simulink model "SS_1029"  (R2014a)
settings: Solver=FixedStepDiscrete  StartTime=0.0  StopTime=5  FixedStep=0.0005  RelTol=1e-3
values from neighbouring files (symbols this model uses):
  APS_High_null = ecucoder_cal(APS_High_null)    [SS.m]
  APS_High_x = ecucoder_cal(APS_High_x)    [SS.m]
  APS_High_y = ecucoder_cal(APS_High_y)    [SS.m]
  APS_Low_null = ecucoder_cal(APS_Low_null)    [SS.m]
  APS_low_x = ecucoder_cal(APS_low_x)    [SS.m]
  APS_low_y = ecucoder_cal(APS_low_y)    [SS.m]
  BrakeSignal_cal = ecucoder_cal(BrakeSignal_cal)    [SS.m]
  CustomReduceFactor_cal = ecucoder_cal(CustomReduceFactor_cal)    [SS.m]
  Differential_cal = ecucoder_cal(Differential_cal)    [SS.m]
  LowSOCWarning_cal = ecucoder_cal(LowSOCWarning_cal)    [SS.m]
  MotorTemperatureHigh_cal = ecucoder_cal(MotorTemperatureHigh_cal)    [SS.m]
  MotorTemperatureLow_cal = ecucoder_cal(MotorTemperatureLow_cal)    [SS.m]
  OilPressure_x = ecucoder_cal(OilPressure_x)    [SS.m]
  OilPressure_y = ecucoder_cal(OilPressure_y)    [SS.m]
  PowerBias_cal = ecucoder_cal(PowerBias_cal)    [SS.m]
  SpeedLimitFactor_x = ecucoder_cal(SpeedLimitFactor_x)    [SS.m]
  SpeedLimitFactor_y = ecucoder_cal(SpeedLimitFactor_y)    [SS.m]
  TorqueLimitNegativ_cal = ecucoder_cal(TorqueLimitNegativ_cal)    [SS.m]
  TorqueLimitPositiv_cal = ecucoder_cal(TorqueLimitPositiv_cal)    [SS.m]
libraries: simulink x101, ec55xxlib x31
(part 1 of 3)
settings Model: Creator=BIT-Battery Group  LastModifiedBy=Administrator
settings OptimizationCC: InlineParams=on  InlineInvariantSignals=on  RollThreshold=9  StateBitsets=on  DataBitsets=on  UseTempVars=on  ZeroExternalMemoryAtStartup=off  ZeroInternalMemoryAtStartup=off  EfficientFloat2IntCast=on  OptimizeModelRefInitCode=on  LifeSpan=Inf
settings DebuggingCC: ConsistencyChecking=warning  MaxConsecutiveZCsMsg=warning  InheritedTsInSrcMsg=none  ModelReferenceExtraNoncontSigs=warning  SimStateOlderReleaseMsg=warning
settings HardwareCC: ProdLargestAtomicInteger=Long  ProdLargestAtomicFloat=Double  ProdIntDivRoundTo=Zero  ProdEndianess=BigEndian  ProdHWDeviceType=Freescale MPC5500
settings RTWCC: SystemTargetFile=ec55xx.tlc  MakeCommand=make_rtw optimized_fixed_point=1  GenerateMakefile=off  TemplateMakefile=ec55xx_lcc.tmf  PostCodeGenCommand=ec55xx_pst_s2(buildInfo)  Description=Target for EC55XX  GenerateReport=on  ProcessScript=ec55xx_make_rtw_hook  IncludeHyperlinkInReport=on  LaunchReport=on
settings CodeAppCC: IgnoreCustomStorageClasses=off
settings STFCustomTargetCC: ModelReferenceCompliant=off  ConcurrentExecutionCompliant=off  IncludeMdlTerminateFcn=off  GeneratePreprocessorConditionals=Use local settings  CombineOutputUpdateFcns=on  SuppressErrorStatus=on  ERTCustomFileBanners=on  SupportContinuousTime=off  SupportNonInlinedSFcns=off  MATLABClassNameForMDSCustomization=Simulink.SoftwareTarget.ERTCustomization  GRTInterface=off  SystemTargetFile=ec55xx.tlc
settings ERTTargetCC: GenerateSampleERTMain=off  ModelReferenceCompliant=off  IncludeMdlTerminateFcn=off  SuppressErrorStatus=on  GenerateASAP2=on  ERTSrcFileBannerTemplate=ec55xx_code_template.cgt  ERTHdrFileBannerTemplate=ec55xx_code_template.cgt  ERTDataSrcFileTemplate=ec55xx_code_template.cgt  ERTDataHdrFileTemplate=ec55xx_code_template.cgt  ERTCustomFileTemplate=ec55xx_file_process.tlc

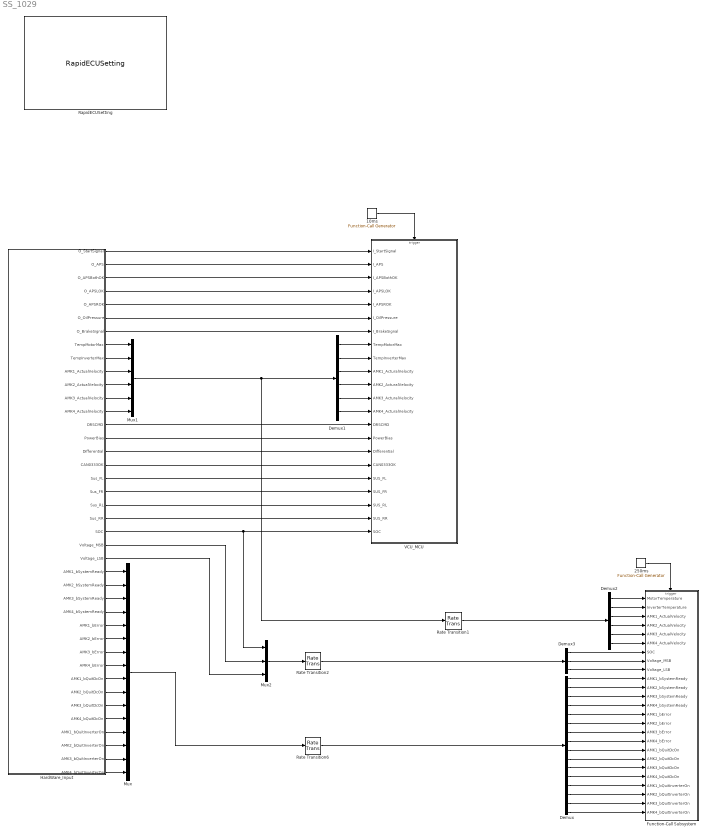
== system SS_1029 ==
  10ms : simulink/Ports & Subsystems/Function-Call Generator  sample_time=0.01  numberOfIterations=1
  250ms : simulink/Ports & Subsystems/Function-Call Generator  sample_time=0.25  numberOfIterations=1
  Demux : Demux  Outputs=16
  Demux1 : Demux  Outputs=6
  Demux2 : Demux  Outputs=6
  Demux3 : Demux  Outputs=3
  Function-Call Subsystem : Subsystem  TreatAsAtomicUnit=on
  HardWare_Input : Subsystem  TreatAsAtomicUnit=on
  Mux : Mux  Inputs=16
  Mux1 : Mux  Inputs=6
  Mux2 : Mux  Inputs=3
  RapidECUSetting : ec55xxlib/RapidECU_U2/RapidECUSetting
  Rate Transition1 : RateTransition  OutPortSampleTime=0.25
  Rate Transition2 : RateTransition  OutPortSampleTime=0.25
  Rate Transition6 : RateTransition  OutPortSampleTime=0.25
  VCU_MCU : Subsystem  TreatAsAtomicUnit=on
  wires:
  HardWare_Input/1(O_StartSignal) -> VCU_MCU/1(I_StartSignal)
  HardWare_Input/5(O_APSROK) -> VCU_MCU/5(I_APSROK)
  HardWare_Input/6(O_OilPressure) -> VCU_MCU/6(I_OilPressure)
  HardWare_Input/4(O_APSLOK) -> VCU_MCU/4(I_APSLOK)
  HardWare_Input/3(O_APSBothOK) -> VCU_MCU/3(I_APSBothOK)
  HardWare_Input/2(O_APS) -> VCU_MCU/2(I_APS)
  10ms/1 -> VCU_MCU/Trigger
  HardWare_Input/7(O_BrakeSignal) -> VCU_MCU/7(I_BrakeSignal)
  250ms/1 -> Function-Call Subsystem/Trigger
  HardWare_Input/22(SOC) -> Mux2/1, VCU_MCU/22(SOC)
  HardWare_Input/14(DRSCMD) -> VCU_MCU/14(DRSCMD)
  HardWare_Input/18(Sus_FL) -> VCU_MCU/18(SUS_FL)
  HardWare_Input/19(Sus_FR) -> VCU_MCU/19("SUS_FR ")
  HardWare_Input/20(Sus_RL) -> VCU_MCU/20(SUS_RL)
  HardWare_Input/21("Sus_RR ") -> VCU_MCU/21(SUS_RR)
  HardWare_Input/15(PowerBias) -> VCU_MCU/15(PowerBias)
  HardWare_Input/16(Differential) -> VCU_MCU/16(Differential)
  HardWare_Input/17(CAN0333OK) -> VCU_MCU/17(CAN0333OK)
  HardWare_Input/27(AMK3_bSystemReady) -> Mux/3
  HardWare_Input/30(AMK2_bError) -> Mux/6
  HardWare_Input/31(AMK3_bError) -> Mux/7
  HardWare_Input/35(AMK3_bQuitDcOn) -> Mux/11
  HardWare_Input/28(AMK4_bSystemReady) -> Mux/4
  HardWare_Input/36(AMK4_bQuitDcOn) -> Mux/12
  HardWare_Input/38(AMK2_bQuitInverterOn) -> Mux/14
  HardWare_Input/39(AMK3_bQuitInverterOn) -> Mux/15
  HardWare_Input/29(AMK1_bError) -> Mux/5
  HardWare_Input/25(AMK1_bSystemReady) -> Mux/1
  HardWare_Input/40(AMK4_bQuitInverterOn) -> Mux/16
  HardWare_Input/26(AMK2_bSystemReady) -> Mux/2
  HardWare_Input/37(AMK1_bQuitInverterOn) -> Mux/13
  HardWare_Input/32(AMK4_bError) -> Mux/8
  HardWare_Input/34(AMK2_bQuitDcOn) -> Mux/10
  HardWare_Input/33(AMK1_bQuitDcOn) -> Mux/9
  Mux/1 -> Rate Transition6/1
  Rate Transition6/1 -> Demux/1
  Demux/1 -> Function-Call Subsystem/10(AMK1_bSystemReady)
  Demux/2 -> Function-Call Subsystem/11(AMK2_bSystemReady)
  Demux/5 -> Function-Call Subsystem/14(AMK1_bError)
  Demux/7 -> Function-Call Subsystem/16(AMK3_bError)
  Demux/10 -> Function-Call Subsystem/19(AMK2_bQuitDcOn)
  Demux/12 -> Function-Call Subsystem/21(AMK4_bQuitDcOn)
  Demux/13 -> Function-Call Subsystem/22(AMK1_bQuitInverterOn)
  Demux/9 -> Function-Call Subsystem/18(AMK1_bQuitDcOn)
  Demux/14 -> Function-Call Subsystem/23(AMK2_bQuitInverterOn)
  Demux/8 -> Function-Call Subsystem/17(AMK4_bError)
  Demux/4 -> Function-Call Subsystem/13(AMK4_bSystemReady)
  Demux/11 -> Function-Call Subsystem/20(AMK3_bQuitDcOn)
  Demux/6 -> Function-Call Subsystem/15(AMK2_bError)
  Demux/15 -> Function-Call Subsystem/24(AMK3_bQuitInverterOn)
  Demux/3 -> Function-Call Subsystem/12(AMK3_bSystemReady)
  Demux/16 -> Function-Call Subsystem/25(AMK4_bQuitInverterOn)
  HardWare_Input/11(AMK2_ActualVelocity) -> Mux1/4
  HardWare_Input/8(TempMotorMax) -> Mux1/1
  HardWare_Input/10(AMK1_ActualVelocity) -> Mux1/3
  HardWare_Input/12(AMK3_ActualVelocity) -> Mux1/5
  HardWare_Input/13(AMK4_ActualVelocity) -> Mux1/6
  HardWare_Input/9(TempInverterMax) -> Mux1/2
  Demux1/6 -> VCU_MCU/13(AMK4_ActuralVelocity)
  Demux1/3 -> VCU_MCU/10(AMK1_ActuralVelocity)
  Demux1/4 -> VCU_MCU/11(AMK2_ActuralVelocity)
  Demux1/5 -> VCU_MCU/12(AMK3_ActuralVelocity)
  Demux1/2 -> VCU_MCU/9(TempInverterMax)
  Demux1/1 -> VCU_MCU/8(TempMotorMax)
  Mux1/1 -> Demux1/1, Rate Transition1/1
  Demux2/5 -> Function-Call Subsystem/5(AMK3_ActualVelocity)
  Demux2/2 -> Function-Call Subsystem/2(InverterTemperature)
  Demux2/3 -> Function-Call Subsystem/3(AMK1_ActualVelocity)
  Demux2/6 -> Function-Call Subsystem/6(AMK4_ActualVelocity)
  Demux2/1 -> Function-Call Subsystem/1(MotorTemperature)
  Demux2/4 -> Function-Call Subsystem/4(AMK2_ActualVelocity)
  Rate Transition1/1 -> Demux2/1
  Mux2/1 -> Rate Transition2/1
  Demux3/3 -> Function-Call Subsystem/9(Voltage_LSB)
  Demux3/1 -> Function-Call Subsystem/7(SOC)
  Demux3/2 -> Function-Call Subsystem/8(Voltage_MSB)
  Rate Transition2/1 -> Demux3/1
  HardWare_Input/23(Voltage_MSB) -> Mux2/2
  HardWare_Input/24(Voltage_LSB) -> Mux2/3

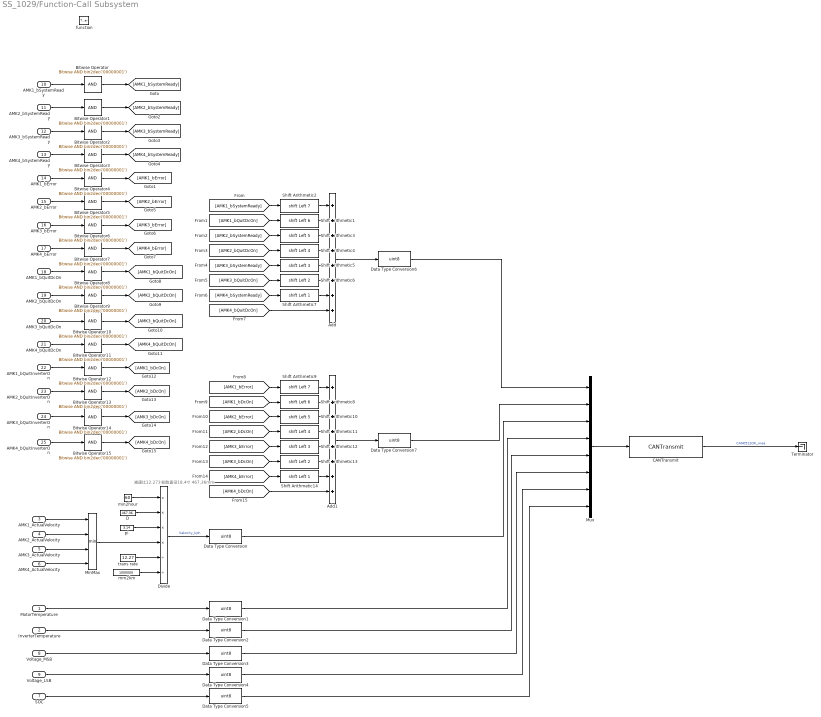
== system SS_1029/Function-Call Subsystem ==
  note: 减速比12.273 轮胎直径18.4寸 467.36mm
  MotorTemperature : Inport
  InverterTemperature : Inport  Port=2
  AMK1_ActualVelocity : Inport  Port=3
  AMK2_ActualVelocity : Inport  Port=4
  AMK3_ActualVelocity : Inport  Port=5
  AMK4_ActualVelocity : Inport  Port=6
  SOC : Inport  Port=7
  Voltage_MSB : Inport  Port=8
  Voltage_LSB : Inport  Port=9
  AMK1_bSystemReady : Inport  Port=10
  AMK2_bSystemReady : Inport  Port=11
  AMK3_bSystemReady : Inport  Port=12
  AMK4_bSystemReady : Inport  Port=13
  AMK1_bError : Inport  Port=14
  AMK2_bError : Inport  Port=15
  AMK3_bError : Inport  Port=16
  AMK4_bError : Inport  Port=17
  AMK1_bQuitDcOn : Inport  Port=18
  AMK2_bQuitDcOn : Inport  Port=19
  AMK3_bQuitDcOn : Inport  Port=20
  AMK4_bQuitDcOn : Inport  Port=21
  AMK1_bQuitInverterOn : Inport  Port=22
  AMK2_bQuitInverterOn : Inport  Port=23
  AMK3_bQuitInverterOn : Inport  Port=24
  AMK4_bQuitInverterOn : Inport  Port=25
  function : TriggerPort  TriggerType=function-call
  Add : Sum  Inputs=++++++++
  Add1 : Sum  Inputs=++++++++
  Bitwise Operator{,1..15} (16 alike) : simulink/Logic and Bit Operations/Bitwise Operator  logicop=AND  UseBitMask=on  BitMask=bin2dec('00000001')  BitMaskRealWorld=Stored Integer
  CANTransmit : ec55xxlib/RapidECU_U2/07CANCommucation/CANTransmit  canmodule=B  canbuffer=15  canmessageid=hex2dec('0512')  canmessagetype=Standard(11-bit ID)  datalength=8  sampletime=-1
  D : Constant  Value=467.36  SampleTime=-1
  Data Type Conversion{,1..7} (8 alike) : DataTypeConversion  OutDataTypeStr=uint8
  Divide : Product  Inputs=****//
  MinMax : MinMax  Inputs=4
  Mux : Mux  Inputs=8
  Shift Arithmetic1 : ArithShift  BitShiftNumber=6  BitShiftDirection=Left
  Shift Arithmetic10 : ArithShift  BitShiftNumber=5  BitShiftDirection=Left
  Shift Arithmetic11 : ArithShift  BitShiftNumber=4  BitShiftDirection=Left
  Shift Arithmetic12 : ArithShift  BitShiftNumber=3  BitShiftDirection=Left
  Shift Arithmetic13 : ArithShift  BitShiftNumber=2  BitShiftDirection=Left
  Shift Arithmetic14 : ArithShift  BitShiftNumber=1  BitShiftDirection=Left
  Shift Arithmetic2 : ArithShift  BitShiftNumber=7  BitShiftDirection=Left
  Shift Arithmetic3 : ArithShift  BitShiftNumber=5  BitShiftDirection=Left
  Shift Arithmetic4 : ArithShift  BitShiftNumber=4  BitShiftDirection=Left
  Shift Arithmetic5 : ArithShift  BitShiftNumber=3  BitShiftDirection=Left
  Shift Arithmetic6 : ArithShift  BitShiftNumber=2  BitShiftDirection=Left
  Shift Arithmetic7 : ArithShift  BitShiftNumber=1  BitShiftDirection=Left
  Shift Arithmetic8 : ArithShift  BitShiftNumber=6  BitShiftDirection=Left
  Shift Arithmetic9 : ArithShift  BitShiftNumber=7  BitShiftDirection=Left
  Terminator : Terminator
  min2hour : Constant  Value=60  SampleTime=-1
  mm2km : Constant  Value=1000000  SampleTime=-1
  pi : Constant  Value=3.14  SampleTime=-1
  trans rate : Constant  Value=12.27  SampleTime=-1
  wires:
  AMK1_ActualVelocity/1 -> MinMax/1
  AMK2_ActualVelocity/1 -> MinMax/2
  AMK3_ActualVelocity/1 -> MinMax/3
  AMK4_ActualVelocity/1 -> MinMax/4
  MinMax/1 -> Divide/4
  min2hour/1 -> Divide/1
  D/1 -> Divide/2
  pi/1 -> Divide/3
  trans rate/1 -> Divide/5
  mm2km/1 -> Divide/6
  Divide/1 -> Data Type Conversion/1  "Velocity_kph"
  MotorTemperature/1 -> Data Type Conversion1/1
  InverterTemperature/1 -> Data Type Conversion2/1
  SOC/1 -> Data Type Conversion5/1
  Voltage_LSB/1 -> Data Type Conversion4/1
  Voltage_MSB/1 -> Data Type Conversion3/1
  AMK1_bSystemReady/1 -> Bitwise Operator/1
  AMK4_bSystemReady/1 -> Bitwise Operator3/1
  AMK3_bSystemReady/1 -> Bitwise Operator2/1
  AMK2_bSystemReady/1 -> Bitwise Operator1/1
  AMK1_bError/1 -> Bitwise Operator4/1
  AMK4_bError/1 -> Bitwise Operator7/1
  AMK3_bError/1 -> Bitwise Operator6/1
  AMK2_bError/1 -> Bitwise Operator5/1
  AMK1_bQuitDcOn/1 -> Bitwise Operator8/1
  AMK2_bQuitDcOn/1 -> Bitwise Operator9/1
  AMK3_bQuitDcOn/1 -> Bitwise Operator10/1
  AMK4_bQuitDcOn/1 -> Bitwise Operator11/1
  AMK1_bQuitInverterOn/1 -> Bitwise Operator12/1
  AMK2_bQuitInverterOn/1 -> Bitwise Operator13/1
  AMK3_bQuitInverterOn/1 -> Bitwise Operator14/1
  AMK4_bQuitInverterOn/1 -> Bitwise Operator15/1
  Bitwise Operator/1 -> [AMK1_bSystemReady]
  Bitwise Operator3/1 -> [AMK4_bSystemReady]
  Bitwise Operator2/1 -> [AMK3_bSystemReady]
  Bitwise Operator1/1 -> [AMK2_bSystemReady]
  Bitwise Operator4/1 -> [AMK1_bError]
  Bitwise Operator7/1 -> [AMK4_bError]
  Bitwise Operator6/1 -> [AMK3_bError]
  Bitwise Operator5/1 -> [AMK2_bError]
  Bitwise Operator8/1 -> [AMK1_bQuitDcOn]
  Bitwise Operator11/1 -> [AMK4_bQuitDcOn]
  Bitwise Operator10/1 -> [AMK3_bQuitDcOn]
  Bitwise Operator9/1 -> [AMK2_bQuitDcOn]
  Bitwise Operator12/1 -> [AMK1_bDcOn]
  Bitwise Operator13/1 -> [AMK2_bDcOn]
  Bitwise Operator14/1 -> [AMK3_bDcOn]
  Bitwise Operator15/1 -> [AMK4_bDcOn]
  [AMK1_bSystemReady] -> Shift Arithmetic2/1
  Shift Arithmetic2/1 -> Add/1
  [AMK1_bQuitDcOn] -> Shift Arithmetic1/1
  Shift Arithmetic1/1 -> Add/2
  [AMK2_bSystemReady] -> Shift Arithmetic3/1
  Shift Arithmetic3/1 -> Add/3
  [AMK2_bQuitDcOn] -> Shift Arithmetic4/1
  Shift Arithmetic4/1 -> Add/4
  [AMK3_bSystemReady] -> Shift Arithmetic5/1
  Shift Arithmetic5/1 -> Add/5
  [AMK3_bQuitDcOn] -> Shift Arithmetic6/1
  Shift Arithmetic6/1 -> Add/6
  [AMK4_bSystemReady] -> Shift Arithmetic7/1
  Shift Arithmetic7/1 -> Add/7
  [AMK4_bQuitDcOn] -> Add/8
  Add/1 -> Data Type Conversion6/1
  [AMK1_bError] -> Shift Arithmetic9/1
  Shift Arithmetic9/1 -> Add1/1
  [AMK1_bDcOn] -> Shift Arithmetic8/1
  Shift Arithmetic8/1 -> Add1/2
  [AMK2_bError] -> Shift Arithmetic10/1
  Shift Arithmetic10/1 -> Add1/3
  [AMK2_bDcOn] -> Shift Arithmetic11/1
  Shift Arithmetic11/1 -> Add1/4
  [AMK3_bError] -> Shift Arithmetic12/1
  Shift Arithmetic12/1 -> Add1/5
  [AMK3_bDcOn] -> Shift Arithmetic13/1
  Shift Arithmetic13/1 -> Add1/6
  [AMK4_bError] -> Shift Arithmetic14/1
  Shift Arithmetic14/1 -> Add1/7
  [AMK4_bDcOn] -> Add1/8
  Add1/1 -> Data Type Conversion7/1
  Data Type Conversion6/1 -> Mux/1
  Data Type Conversion7/1 -> Mux/2
  Data Type Conversion/1 -> Mux/3
  Data Type Conversion1/1 -> Mux/4
  Data Type Conversion2/1 -> Mux/5
  Data Type Conversion3/1 -> Mux/6
  Data Type Conversion4/1 -> Mux/7
  Data Type Conversion5/1 -> Mux/8
  Mux/1 -> CANTransmit/1
  CANTransmit/1 -> Terminator/1  "CAN0512OK_mea"

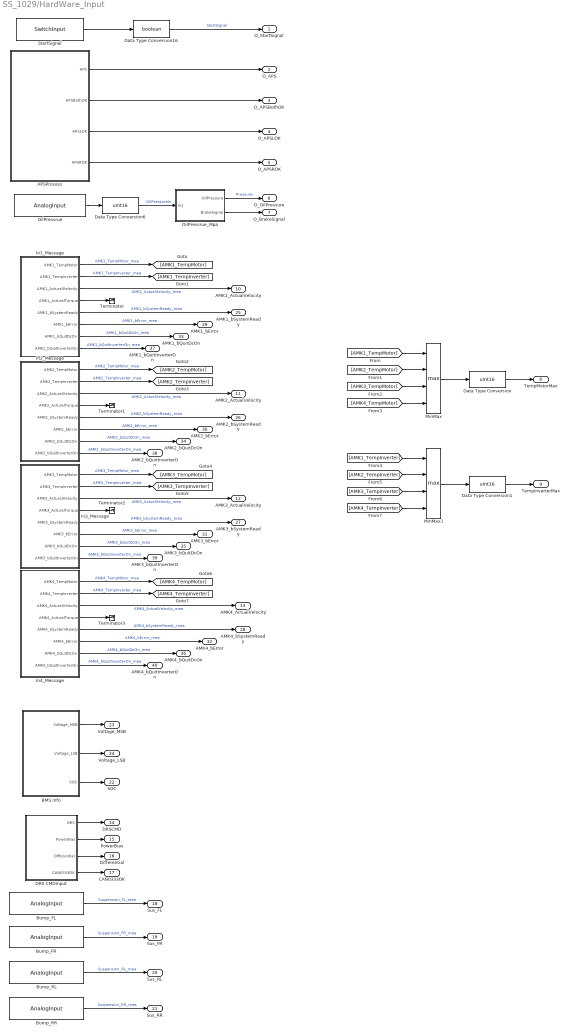
== system SS_1029/HardWare_Input ==
  APSProcess : Subsystem
  BMS Info : Subsystem  TreatAsAtomicUnit=on
  Bump_FL : ec55xxlib/RapidECU_U2/02AnalogInput/AnalogInput  channel=53: I_AN14_5V  sampletime=-1
  Bump_FR : ec55xxlib/RapidECU_U2/02AnalogInput/AnalogInput  channel=54: I_AN15_5V  sampletime=-1
  Bump_RL : ec55xxlib/RapidECU_U2/02AnalogInput/AnalogInput  channel=55: I_AN16_5V  sampletime=-1
  Bump_RR : ec55xxlib/RapidECU_U2/02AnalogInput/AnalogInput  channel=56: I_AN17_5V  sampletime=-1
  DRS CMDInput : Subsystem  TreatAsAtomicUnit=on
  Data Type Conversion : DataTypeConversion  OutDataTypeStr=uint16
  Data Type Conversion1 : DataTypeConversion  OutDataTypeStr=uint16
  Data Type Conversion16 : DataTypeConversion  OutDataTypeStr=boolean
  Data Type Conversion6 : DataTypeConversion  OutDataTypeStr=uint16
  In1_Message : Subsystem
  In2_Message : Subsystem
  In3_Message : Subsystem
  In4_Message : Subsystem
  MinMax : MinMax  Function=max  Inputs=4
  MinMax1 : MinMax  Function=max  Inputs=4
  OilPressrue : ec55xxlib/RapidECU_U1/02AnalogInput/AnalogInput  channel=73: I_AN19_5V  sampletime=-1
  OilPressrue_Mpa : Subsystem
  StartSignal : ec55xxlib/RapidECU_U2/01SwitchInput/SwitchInput  channel=44: I_SW11_H  sampletime=-1
  Terminator{,1..3} (4 alike) : Terminator
  O_StartSignal : Outport
  O_APS : Outport  Port=2
  O_APSBothOK : Outport  Port=3
  O_APSLOK : Outport  Port=4
  O_APSROK : Outport  Port=5
  O_OilPressure : Outport  Port=6
  O_BrakeSignal : Outport  Port=7
  TempMotorMax : Outport  Port=8
  TempInverterMax : Outport  Port=9
  AMK1_ActualVelocity : Outport  Port=10
  AMK2_ActualVelocity : Outport  Port=11
  AMK3_ActualVelocity : Outport  Port=12
  AMK4_ActualVelocity : Outport  Port=13
  DRSCMD : Outport  Port=14
  PowerBias : Outport  Port=15
  Differential : Outport  Port=16
  CAN0333OK : Outport  Port=17
  Sus_FL : Outport  Port=18
  Sus_FR : Outport  Port=19
  Sus_RL : Outport  Port=20
  "Sus_RR " : Outport  Port=21
  SOC : Outport  Port=22
  Voltage_MSB : Outport  Port=23
  Voltage_LSB : Outport  Port=24
  AMK1_bSystemReady : Outport  Port=25
  AMK2_bSystemReady : Outport  Port=26
  AMK3_bSystemReady : Outport  Port=27
  AMK4_bSystemReady : Outport  Port=28
  AMK1_bError : Outport  Port=29
  AMK2_bError : Outport  Port=30
  AMK3_bError : Outport  Port=31
  AMK4_bError : Outport  Port=32
  AMK1_bQuitDcOn : Outport  Port=33
  AMK2_bQuitDcOn : Outport  Port=34
  AMK3_bQuitDcOn : Outport  Port=35
  AMK4_bQuitDcOn : Outport  Port=36
  AMK1_bQuitInverterOn : Outport  Port=37
  AMK2_bQuitInverterOn : Outport  Port=38
  AMK3_bQuitInverterOn : Outport  Port=39
  AMK4_bQuitInverterOn : Outport  Port=40
  wires:
  OilPressrue_Mpa/1(OilPressure) -> O_OilPressure/1  "Pressure"
  Data Type Conversion16/1 -> O_StartSignal/1  "StartSignal"
  StartSignal/1 -> Data Type Conversion16/1
  Data Type Conversion6/1 -> OilPressrue_Mpa/1(In1)  "OilPressureIn"
  OilPressrue/1 -> Data Type Conversion6/1
  APSProcess/1(APS) -> O_APS/1
  APSProcess/2(APSBothOK) -> O_APSBothOK/1
  APSProcess/3(APSLOK) -> O_APSLOK/1
  APSProcess/4(APSROK) -> O_APSROK/1
  In1_Message/1(AMK1_TempMotor) -> [AMK1_TempMotor]  "AMK1_TempMotor_mea"
  In1_Message/2(AMK1_TempInverter) -> [AMK1_TempInverter]  "AMK1_TempInverter_mea"
  In2_Message/1(AMK2_TempMotor) -> [AMK2_TempMotor]  "AMK2_TempMotor_mea"
  In2_Message/2(AMK2_TempInverter) -> [AMK2_TempInverter]  "AMK2_TempInverter_mea"
  In3_Message/1(AMK3_TempMotor) -> [AMK3_TempMotor]  "AMK3_TempMotor_mea"
  In3_Message/2(AMK3_TempInverter) -> [AMK3_TempInverter]  "AMK3_TempInverter_mea"
  In4_Message/1(AMK4_TempMotor) -> [AMK4_TempMotor]  "AMK4_TempMotor_mea"
  In4_Message/2(AMK4_TempInverter) -> [AMK4_TempInverter]  "AMK4_TempInverter_mea"
  [AMK1_TempMotor] -> MinMax/1
  [AMK3_TempMotor] -> MinMax/3
  [AMK2_TempMotor] -> MinMax/2
  [AMK4_TempMotor] -> MinMax/4
  [AMK1_TempInverter] -> MinMax1/1
  [AMK2_TempInverter] -> MinMax1/2
  [AMK4_TempInverter] -> MinMax1/4
  [AMK3_TempInverter] -> MinMax1/3
  MinMax/1 -> Data Type Conversion/1
  MinMax1/1 -> Data Type Conversion1/1
  OilPressrue_Mpa/2(BrakeSignal) -> O_BrakeSignal/1
  In1_Message/4(AMK1_ActuralTorque) -> Terminator/1
  In2_Message/4(AMK2_ActuralTorque) -> Terminator1/1
  In3_Message/4(AMK3_ActuralTorque) -> Terminator2/1
  In4_Message/4(AMK4_ActuralTorque) -> Terminator3/1
  In1_Message/3(AMK1_ActuralVelocity) -> AMK1_ActualVelocity/1  "AMK1_ActualVelocity_mea"
  In2_Message/3(AMK2_ActuralVelocity) -> AMK2_ActualVelocity/1  "AMK2_ActualVelocity_mea"
  In3_Message/3(AMK3_ActuralVelocity) -> AMK3_ActualVelocity/1  "AMK3_ActualVelocity_mea"
  In4_Message/3(AMK4_ActuralVelocity) -> AMK4_ActualVelocity/1  "AMK4_ActualVelocity_mea"
  In4_Message/5(AMK4_bSystemReady) -> AMK4_bSystemReady/1  "AMK4_bSystemReady_mea"
  In3_Message/5(AMK3_bSystemReady) -> AMK3_bSystemReady/1  "AMK3_bSystemReady_mea"
  In2_Message/5(AMK2_bSystemReady) -> AMK2_bSystemReady/1  "AMK2_bSystemReady_mea"
  In1_Message/5(AMK1_bSystemReady) -> AMK1_bSystemReady/1  "AMK1_bSystemReady_mea"
  In1_Message/6(AMK1_bError) -> AMK1_bError/1  "AMK1_bError_mea"
  In2_Message/6(AMK2_bError) -> AMK2_bError/1  "AMK2_bError_mea"
  In3_Message/6(AMK3_bError) -> AMK3_bError/1  "AMK3_bError_mea"
  In4_Message/6(AMK4_bError) -> AMK4_bError/1  "AMK4_bError_mea"
  In3_Message/7(AMK3_bQuitDcOn) -> AMK3_bQuitDcOn/1  "AMK3_bQuitDcOn_mea"
  In4_Message/7(AMK4_bQuitDcOn) -> AMK4_bQuitDcOn/1  "AMK4_bQuitDcOn_mea"
  In2_Message/7(AMK2_bQuitDcOn) -> AMK2_bQuitDcOn/1  "AMK2_bQuitDcOn_mea"
  In1_Message/7(AMK1_bQuitDcOn) -> AMK1_bQuitDcOn/1  "AMK1_bQuitDcOn_mea"
  In1_Message/8(AMK1_bQuitInverterOn) -> AMK1_bQuitInverterOn/1  "AMK1_bQuitInverterOn_mea"
  In2_Message/8(AMK2_bQuitInverterOn) -> AMK2_bQuitInverterOn/1  "AMK2_bQuitInverterOn_mea"
  In3_Message/8(AMK3_bQuitInverterOn) -> AMK3_bQuitInverterOn/1  "AMK3_bQuitInverterOn_mea"
  In4_Message/8(AMK4_bQuitInverterOn) -> AMK4_bQuitInverterOn/1  "AMK4_bQuitInverterOn_mea"
  BMS Info/1(Voltage_MSB) -> Voltage_MSB/1
  BMS Info/2(Voltage_LSB) -> Voltage_LSB/1
  BMS Info/3(SOC) -> SOC/1
  DRS CMDInput/1(DRS) -> DRSCMD/1
  Bump_FL/1 -> Sus_FL/1  "Suspension_FL_mea"
  Bump_FR/1 -> Sus_FR/1  "Suspension_FR_mea"
  Bump_RL/1 -> Sus_RL/1  "Suspension_RL_mea"
  Bump_RR/1 -> "Sus_RR "/1  "Suspension_RR_mea"
  DRS CMDInput/2(PowerBias) -> PowerBias/1
  DRS CMDInput/3(Differential) -> Differential/1
  DRS CMDInput/4(CAN0333OK) -> CAN0333OK/1
  Data Type Conversion/1 -> TempMotorMax/1
  Data Type Conversion1/1 -> TempInverterMax/1

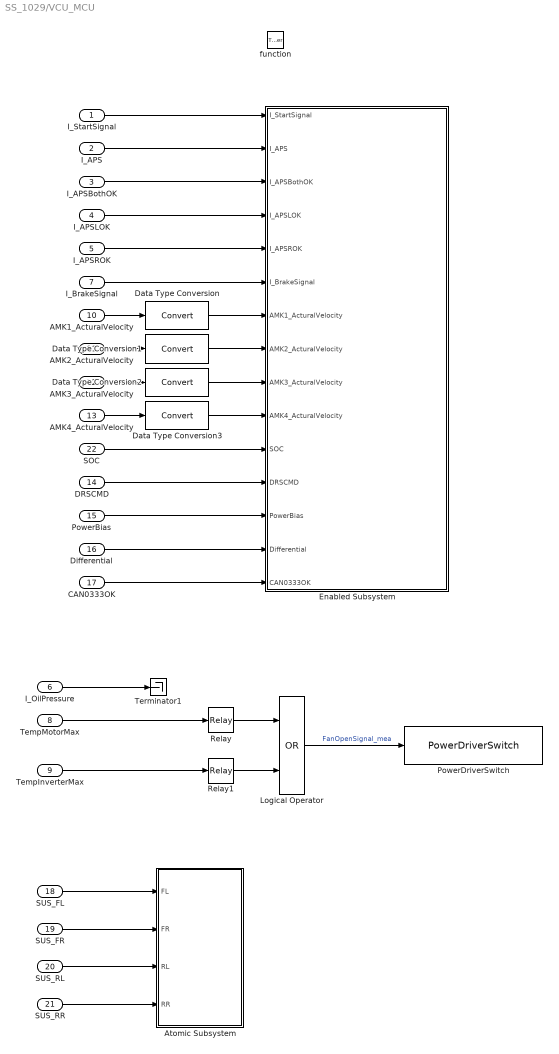
== system SS_1029/VCU_MCU ==
  I_StartSignal : Inport
  I_APS : Inport  Port=2
  I_APSBothOK : Inport  Port=3
  I_APSLOK : Inport  Port=4
  I_APSROK : Inport  Port=5
  I_OilPressure : Inport  Port=6
  I_BrakeSignal : Inport  Port=7
  TempMotorMax : Inport  Port=8
  TempInverterMax : Inport  Port=9
  AMK1_ActuralVelocity : Inport  Port=10
  AMK2_ActuralVelocity : Inport  Port=11
  AMK3_ActuralVelocity : Inport  Port=12
  AMK4_ActuralVelocity : Inport  Port=13
  DRSCMD : Inport  Port=14
  PowerBias : Inport  Port=15
  Differential : Inport  Port=16
  CAN0333OK : Inport  Port=17
  SUS_FL : Inport  Port=18
  "SUS_FR " : Inport  Port=19
  SUS_RL : Inport  Port=20
  SUS_RR : Inport  Port=21
  SOC : Inport  Port=22
  function : TriggerPort  TriggerType=function-call
  Atomic Subsystem : Subsystem  TreatAsAtomicUnit=on
  Data Type Conversion{,1..3} (4 alike) : DataTypeConversion
  Enabled Subsystem : Subsystem  TreatAsAtomicUnit=on
  Logical Operator : Logic  Operator=OR  AllPortsSameDT=off  OutDataTypeStr=boolean
  PowerDriverSwitch : ec55xxlib/RapidECU_U2/04PowerDriverSwitch/PowerDriverSwitch  channel=117: O_PWM11_HS2A9  sampletime=-1
  Relay : Relay  OnSwitchValue=MotorTemperatureHigh_cal  OffSwitchValue=MotorTemperatureLow_cal
  Relay1 : Relay  OnSwitchValue=MotorTemperatureHigh_cal  OffSwitchValue=MotorTemperatureLow_cal
  Terminator1 : Terminator
  wires:
  I_StartSignal/1 -> Enabled Subsystem/1(I_StartSignal)
  I_APSBothOK/1 -> Enabled Subsystem/3(I_APSBothOK)
  I_APSROK/1 -> Enabled Subsystem/5(I_APSROK)
  I_APSLOK/1 -> Enabled Subsystem/4(I_APSLOK)
  I_OilPressure/1 -> Terminator1/1
  TempMotorMax/1 -> Relay/1
  TempInverterMax/1 -> Relay1/1
  I_APS/1 -> Enabled Subsystem/2(I_APS)
  I_BrakeSignal/1 -> Enabled Subsystem/6(I_BrakeSignal)
  Relay1/1 -> Logical Operator/2
  Relay/1 -> Logical Operator/1
  Logical Operator/1 -> PowerDriverSwitch/1  "FanOpenSignal_mea"
  AMK1_ActuralVelocity/1 -> Data Type Conversion/1
  AMK2_ActuralVelocity/1 -> Data Type Conversion1/1
  AMK3_ActuralVelocity/1 -> Data Type Conversion2/1
  AMK4_ActuralVelocity/1 -> Data Type Conversion3/1
  Data Type Conversion/1 -> Enabled Subsystem/7(AMK1_ActuralVelocity)
  Data Type Conversion1/1 -> Enabled Subsystem/8(AMK2_ActuralVelocity)
  Data Type Conversion2/1 -> Enabled Subsystem/9(AMK3_ActuralVelocity)
  Data Type Conversion3/1 -> Enabled Subsystem/10(AMK4_ActuralVelocity)
  SOC/1 -> Enabled Subsystem/11(SOC)
  DRSCMD/1 -> Enabled Subsystem/12(DRSCMD)
  SUS_FL/1 -> Atomic Subsystem/1(FL)
  "SUS_FR "/1 -> Atomic Subsystem/2(FR)
  SUS_RL/1 -> Atomic Subsystem/3(RL)
  SUS_RR/1 -> Atomic Subsystem/4(RR)
  PowerBias/1 -> Enabled Subsystem/13(PowerBias)
  Differential/1 -> Enabled Subsystem/14(Differential)
  CAN0333OK/1 -> Enabled Subsystem/15(CAN0333OK)

== system SS_1029/HardWare_Input/APSProcess ==
  1-D Lookup Table : Lookup_n-D  NumberOfTableDimensions=1  BreakpointsForDimension1=APS_low_x  BreakpointsForDimension1DataTypeStr=single  Table=APS_low_y  TableDataTypeStr=single  ExtrapMethod=Clip  InternalRulePriority=Speed  OutDataTypeStr=single  RndMeth=Simplest  InputSameDT=on
  1-D Lookup Table1 : Lookup_n-D  NumberOfTableDimensions=1  BreakpointsForDimension1=APS_High_x  BreakpointsForDimension1DataTypeStr=single  Table=APS_High_y  TableDataTypeStr=single  ExtrapMethod=Clip  InternalRulePriority=Speed  OutDataTypeStr=single  RndMeth=Simplest  InputSameDT=on
  APS_High : ec55xxlib/RapidECU_U1/02AnalogInput/AnalogInput  channel=71: I_AN18_5V  sampletime=-1
  APS_Low : ec55xxlib/RapidECU_U1/02AnalogInput/AnalogInput  channel=52: I_AN13_5V  sampletime=-1
  Abs : Abs
  Add2 : Sum  AccumDataTypeStr=single
  Add3 : Sum  Inputs=+-  AccumDataTypeStr=single
  Compare To Constant : simulink/Logic and Bit Operations/Compare To Constant  relop=<=  const=5  OutDataTypeStr=boolean
  Constant6 : Constant
  Constant7 : Constant  Value=0
  Constant8 : Constant
  Constant9 : Constant  Value=0
  Data Type Conversion7 : DataTypeConversion  OutDataTypeStr=uint16
  Data Type Conversion8 : DataTypeConversion  OutDataTypeStr=uint16
  Gain1 : Gain  Gain=0.5  OutDataTypeStr=single
  Saturation : Saturate  UpperLimit=2000  LowerLimit=0
  Switch1 : Switch  Criteria=u2 > Threshold  Threshold=APS_Low_null  OutDataTypeStr=uint8
  Switch2 : Switch  Criteria=u2 > Threshold  Threshold=APS_High_null  OutDataTypeStr=uint8
  Terminator : Terminator
  Terminator1 : Terminator
  APS : Outport
  APSBothOK : Outport  Port=2
  APSLOK : Outport  Port=3
  APSROK : Outport  Port=4
  wires:
  Switch2/1 -> APSROK/1  "APSROK_mea"
  Constant9/1 -> Switch2/3
  Constant8/1 -> Switch2/1
  Switch1/1 -> APSLOK/1  "APSLOK_mea"
  Constant7/1 -> Switch1/3
  Constant6/1 -> Switch1/1
  Compare To Constant/1 -> APSBothOK/1  "APSBothOK_mea"
  Abs/1 -> Compare To Constant/1
  Add3/1 -> Abs/1
  Saturation/1 -> APS/1
  Add2/1 -> Gain1/1
  1-D Lookup Table1/1 -> Add3/1, Add2/2, Terminator1/1  "APSHigh_pct"
  1-D Lookup Table/1 -> Add2/1, Terminator/1, Add3/2  "APSLow_pct"
  Data Type Conversion8/1 -> 1-D Lookup Table1/1, Switch2/2  "APS_High"
  Data Type Conversion7/1 -> 1-D Lookup Table/1, Switch1/2  "APS_Low"
  APS_High/1 -> Data Type Conversion8/1
  APS_Low/1 -> Data Type Conversion7/1
  Gain1/1 -> Saturation/1

== system SS_1029/HardWare_Input/BMS Info ==
  CANReceive : ec55xxlib/RapidECU_U2/07CANCommucation/CANReceive  canmodule=B  canbuffer=30  canmessageid=hex2dec('186040F3')  canmessagetype=Extended(29-bit ID)  datalength=8  sampletime=-1
  Subsystem : Subsystem
  Terminator : Terminator
  Terminator1 : Terminator
  Voltage_MSB : Outport
  Voltage_LSB : Outport  Port=2
  SOC : Outport  Port=3
  wires:
  CANReceive/5 -> Terminator/1
  CANReceive/3 -> Terminator1/1
  CANReceive/2 -> Subsystem/1("Enable ")  "BMSCANOK_mea"
  CANReceive/1 -> Subsystem/Trigger
  CANReceive/4 -> Subsystem/2(CANMsg)
  Subsystem/1(Voltage_MSB) -> Voltage_MSB/1
  Subsystem/2(Voltage_LSB) -> Voltage_LSB/1
  Subsystem/3(SOC) -> SOC/1

== system SS_1029/HardWare_Input/DRS CMDInput ==
  CANReceive : ec55xxlib/RapidECU_U2/07CANCommucation/CANReceive  canmodule=B  canbuffer=36  canmessageid=hex2dec('0333')  canmessagetype=Standard(11-bit ID)  datalength=8  sampletime=-1
  Subsystem : Subsystem
  Terminator2 : Terminator
  Terminator3 : Terminator
  DRS : Outport
  PowerBias : Outport  Port=2
  Differential : Outport  Port=3
  CAN0333OK : Outport  Port=4
  wires:
  CANReceive/1 -> Subsystem/Trigger
  CANReceive/2 -> CAN0333OK/1, Subsystem/1(Enable)  "DRSCANOK_mea"
  CANReceive/3 -> Terminator2/1
  CANReceive/5 -> Terminator3/1
  CANReceive/4 -> Subsystem/2(CANMsg)
  Subsystem/1(DRS) -> DRS/1
  Subsystem/2(PowerBias) -> PowerBias/1
  Subsystem/3(Differential) -> Differential/1

== system SS_1029/HardWare_Input/In1_Message ==
  CANReceive : ec55xxlib/RapidECU_U2/07CANCommucation/CANReceive  canmodule=A  canbuffer=0  canmessageid=hex2dec('0283')  canmessagetype=Standard(11-bit ID)  datalength=8  sampletime=-1
  CANReceive1 : ec55xxlib/RapidECU_U2/07CANCommucation/CANReceive  canmodule=A  canbuffer=1  canmessageid=hex2dec('0285')  canmessagetype=Standard(11-bit ID)  datalength=8  sampletime=-1
  Function-Call Subsystem : Subsystem  TreatAsAtomicUnit=on
  Function-Call Subsystem1 : Subsystem  TreatAsAtomicUnit=on
  Terminator{1..2,4..5} (4 alike) : Terminator
  AMK1_TempMotor : Outport
  AMK1_TempInverter : Outport  Port=2
  AMK1_ActuralVelocity : Outport  Port=3
  AMK1_ActuralTorque : Outport  Port=4
  AMK1_bSystemReady : Outport  Port=5
  AMK1_bError : Outport  Port=6
  AMK1_bQuitDcOn : Outport  Port=7
  AMK1_bQuitInverterOn : Outport  Port=8
  wires:
  CANReceive/2 -> Function-Call Subsystem/1(Enable)
  CANReceive/3 -> Terminator1/1
  CANReceive/5 -> Terminator2/1
  CANReceive/1 -> Function-Call Subsystem/Trigger
  CANReceive/4 -> Function-Call Subsystem/2(CANMsg)
  CANReceive1/1 -> Function-Call Subsystem1/Trigger
  CANReceive1/4 -> Function-Call Subsystem1/2(CANMsg)
  CANReceive1/2 -> Function-Call Subsystem1/1(Enable)
  CANReceive1/3 -> Terminator4/1
  CANReceive1/5 -> Terminator5/1
  Function-Call Subsystem/1(AMK_ActuralVelocity) -> AMK1_ActuralVelocity/1
  Function-Call Subsystem/2(AMK_ActuralTorque) -> AMK1_ActuralTorque/1
  Function-Call Subsystem1/1(AMK_TempMotor) -> AMK1_TempMotor/1
  Function-Call Subsystem1/2(AMK_TempInverter) -> AMK1_TempInverter/1
  Function-Call Subsystem/3(AMK_bSystemReady) -> AMK1_bSystemReady/1
  Function-Call Subsystem/4(AMK_bError) -> AMK1_bError/1
  Function-Call Subsystem/5(AMK_bQuitDcOn) -> AMK1_bQuitDcOn/1
  Function-Call Subsystem/6("AMK_bQuitInverterOn ") -> AMK1_bQuitInverterOn/1

== system SS_1029/HardWare_Input/In2_Message ==
  CANReceive2 : ec55xxlib/RapidECU_U2/07CANCommucation/CANReceive  canmodule=A  canbuffer=2  canmessageid=hex2dec('0284')  canmessagetype=Standard(11-bit ID)  datalength=8  sampletime=-1
  CANReceive3 : ec55xxlib/RapidECU_U2/07CANCommucation/CANReceive  canmodule=A  canbuffer=3  canmessageid=hex2dec('0286')  canmessagetype=Standard(11-bit ID)  datalength=8  sampletime=-1
  Function-Call Subsystem : Subsystem  TreatAsAtomicUnit=on
  Function-Call Subsystem1 : Subsystem  TreatAsAtomicUnit=on
  Terminator{1..2,4..5} (4 alike) : Terminator
  AMK2_TempMotor : Outport
  AMK2_TempInverter : Outport  Port=2
  AMK2_ActuralVelocity : Outport  Port=3
  AMK2_ActuralTorque : Outport  Port=4
  AMK2_bSystemReady : Outport  Port=5
  AMK2_bError : Outport  Port=6
  AMK2_bQuitDcOn : Outport  Port=7
  AMK2_bQuitInverterOn : Outport  Port=8
  wires:
  CANReceive2/3 -> Terminator1/1
  CANReceive2/5 -> Terminator2/1
  CANReceive3/3 -> Terminator4/1
  CANReceive3/5 -> Terminator5/1
  CANReceive2/2 -> Function-Call Subsystem/1(Enable)
  CANReceive2/1 -> Function-Call Subsystem/Trigger
  CANReceive2/4 -> Function-Call Subsystem/2(CANMsg)
  CANReceive3/1 -> Function-Call Subsystem1/Trigger
  CANReceive3/4 -> Function-Call Subsystem1/2(CANMsg)
  CANReceive3/2 -> Function-Call Subsystem1/1(Enable)
  Function-Call Subsystem/1(AMK_ActuralVelocity) -> AMK2_ActuralVelocity/1
  Function-Call Subsystem/2(AMK_ActuralTorque) -> AMK2_ActuralTorque/1
  Function-Call Subsystem1/1(AMK_TempMotor) -> AMK2_TempMotor/1
  Function-Call Subsystem1/2(AMK_TempInverter) -> AMK2_TempInverter/1
  Function-Call Subsystem/3(AMK_bSystemReady) -> AMK2_bSystemReady/1
  Function-Call Subsystem/4(AMK_bError) -> AMK2_bError/1
  Function-Call Subsystem/5(AMK_bQuitDcOn) -> AMK2_bQuitDcOn/1
  Function-Call Subsystem/6("AMK_bQuitInverterOn ") -> AMK2_bQuitInverterOn/1

== system SS_1029/HardWare_Input/In3_Message ==
  CANReceive2 : ec55xxlib/RapidECU_U2/07CANCommucation/CANReceive  canmodule=A  canbuffer=4  canmessageid=hex2dec('0287')  canmessagetype=Standard(11-bit ID)  datalength=8  sampletime=-1
  CANReceive3 : ec55xxlib/RapidECU_U2/07CANCommucation/CANReceive  canmodule=A  canbuffer=5  canmessageid=hex2dec('0289')  canmessagetype=Standard(11-bit ID)  datalength=8  sampletime=-1
  Function-Call Subsystem : Subsystem  TreatAsAtomicUnit=on
  Function-Call Subsystem1 : Subsystem  TreatAsAtomicUnit=on
  Terminator{1..2,4..5} (4 alike) : Terminator
  AMK3_TempMotor : Outport
  AMK3_TempInverter : Outport  Port=2
  AMK3_ActuralVelocity : Outport  Port=3
  AMK3_ActuralTorque : Outport  Port=4
  AMK3_bSystemReady : Outport  Port=5
  AMK3_bError : Outport  Port=6
  AMK3_bQuitDcOn : Outport  Port=7
  AMK3_bQuitInverterOn : Outport  Port=8
  wires:
  CANReceive2/3 -> Terminator1/1
  CANReceive2/5 -> Terminator2/1
  CANReceive3/3 -> Terminator4/1
  CANReceive3/5 -> Terminator5/1
  CANReceive2/2 -> Function-Call Subsystem/1(Enable)
  CANReceive2/1 -> Function-Call Subsystem/Trigger
  CANReceive2/4 -> Function-Call Subsystem/2(CANMsg)
  CANReceive3/1 -> Function-Call Subsystem1/Trigger
  CANReceive3/4 -> Function-Call Subsystem1/2(CANMsg)
  Function-Call Subsystem/1(AMK_ActuralVelocity) -> AMK3_ActuralVelocity/1
  Function-Call Subsystem/2(AMK_ActuralTorque) -> AMK3_ActuralTorque/1
  Function-Call Subsystem1/1(AMK_TempMotor) -> AMK3_TempMotor/1
  Function-Call Subsystem1/2(AMK_TempInverter) -> AMK3_TempInverter/1
  Function-Call Subsystem/3(AMK_bSystemReady) -> AMK3_bSystemReady/1
  Function-Call Subsystem/4(AMK_bError) -> AMK3_bError/1
  Function-Call Subsystem/5(AMK_bQuitDcOn) -> AMK3_bQuitDcOn/1
  Function-Call Subsystem/6("AMK_bQuitInverterOn ") -> AMK3_bQuitInverterOn/1
  CANReceive3/2 -> Function-Call Subsystem1/1(Enable)

== system SS_1029/HardWare_Input/In4_Message ==
  CANReceive2 : ec55xxlib/RapidECU_U2/07CANCommucation/CANReceive  canmodule=A  canbuffer=6  canmessageid=hex2dec('0288')  canmessagetype=Standard(11-bit ID)  datalength=8  sampletime=-1
  CANReceive3 : ec55xxlib/RapidECU_U2/07CANCommucation/CANReceive  canmodule=A  canbuffer=7  canmessageid=hex2dec('028A')  canmessagetype=Standard(11-bit ID)  datalength=8  sampletime=-1
  Function-Call Subsystem : Subsystem  TreatAsAtomicUnit=on
  Function-Call Subsystem1 : Subsystem  TreatAsAtomicUnit=on
  Terminator{1..2,4..5} (4 alike) : Terminator
  AMK4_TempMotor : Outport
  AMK4_TempInverter : Outport  Port=2
  AMK4_ActuralVelocity : Outport  Port=3
  AMK4_ActuralTorque : Outport  Port=4
  AMK4_bSystemReady : Outport  Port=5
  AMK4_bError : Outport  Port=6
  AMK4_bQuitDcOn : Outport  Port=7
  AMK4_bQuitInverterOn : Outport  Port=8
  wires:
  CANReceive2/3 -> Terminator1/1
  CANReceive2/5 -> Terminator2/1
  CANReceive3/3 -> Terminator4/1
  CANReceive3/5 -> Terminator5/1
  CANReceive2/2 -> Function-Call Subsystem/1(Enable)
  CANReceive2/1 -> Function-Call Subsystem/Trigger
  CANReceive2/4 -> Function-Call Subsystem/2(CANMsg)
  CANReceive3/1 -> Function-Call Subsystem1/Trigger
  CANReceive3/4 -> Function-Call Subsystem1/2(CANMsg)
  CANReceive3/2 -> Function-Call Subsystem1/1(Enable)
  Function-Call Subsystem/1(AMK_ActuralVelocity) -> AMK4_ActuralVelocity/1
  Function-Call Subsystem/2(AMK_ActuralTorque) -> AMK4_ActuralTorque/1
  Function-Call Subsystem1/1(AMK_TempMotor) -> AMK4_TempMotor/1
  Function-Call Subsystem1/2(AMK_TempInverter) -> AMK4_TempInverter/1
  Function-Call Subsystem/3(AMK_bSystemReady) -> AMK4_bSystemReady/1
  Function-Call Subsystem/4(AMK_bError) -> AMK4_bError/1
  Function-Call Subsystem/5(AMK_bQuitDcOn) -> AMK4_bQuitDcOn/1
  Function-Call Subsystem/6("AMK_bQuitInverterOn ") -> AMK4_bQuitInverterOn/1

== system SS_1029/HardWare_Input/OilPressrue_Mpa ==
  In1 : Inport
  1-D Lookup Table : Lookup_n-D  NumberOfTableDimensions=1  BreakpointsForDimension1=OilPressure_x  BreakpointsForDimension1DataTypeStr=int16  Table=OilPressure_y  TableDataTypeStr=int16  ExtrapMethod=Clip  InternalRulePriority=Speed  OutDataTypeStr=uint8  RndMeth=Simplest  InputSameDT=on
  Compare To Constant : simulink/Logic and Bit Operations/Compare To Constant  relop=>=  const=BrakeSignal_cal  OutDataTypeStr=boolean
  OilPressure : Outport
  BrakeSignal : Outport  Port=2
  wires:
  1-D Lookup Table/1 -> OilPressure/1
  In1/1 -> 1-D Lookup Table/1, Compare To Constant/1
  Compare To Constant/1 -> BrakeSignal/1  "BrakeSignal_mea"

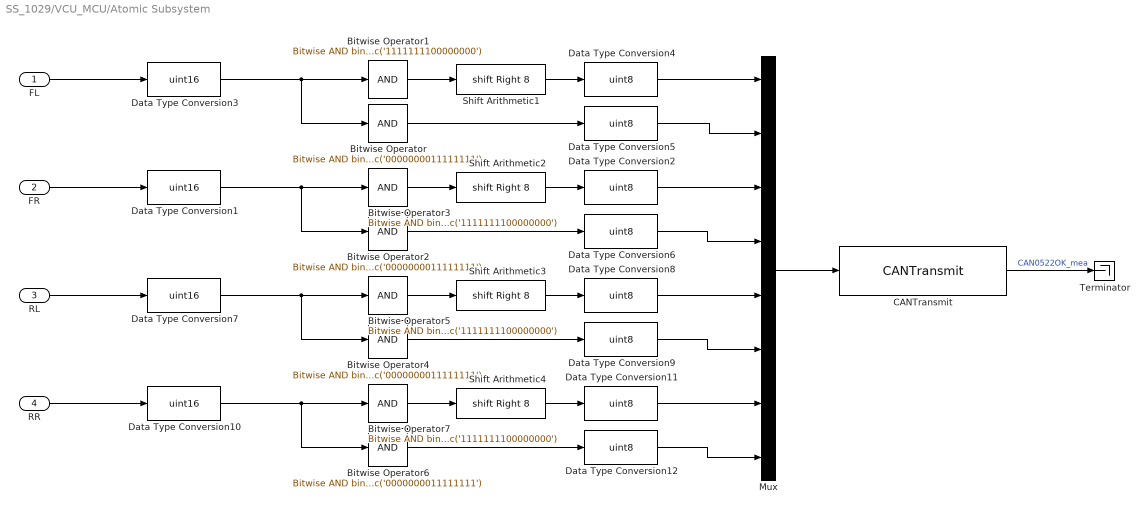
== system SS_1029/VCU_MCU/Atomic Subsystem ==
  FL : Inport
  FR : Inport  Port=2
  RL : Inport  Port=3
  RR : Inport  Port=4
  Bitwise Operator{,2,4,6} (4 alike) : simulink/Logic and Bit Operations/Bitwise Operator  logicop=AND  UseBitMask=on  BitMask=bin2dec('0000000011111111')  BitMaskRealWorld=Stored Integer
  Bitwise Operator{1,3,5,7} (4 alike) : simulink/Logic and Bit Operations/Bitwise Operator  logicop=AND  UseBitMask=on  BitMask=bin2dec('1111111100000000')  BitMaskRealWorld=Stored Integer
  CANTransmit : ec55xxlib/RapidECU_U2/07CANCommucation/CANTransmit  canmodule=B  canbuffer=61  canmessageid=hex2dec('0522')  canmessagetype=Standard(11-bit ID)  datalength=8  sampletime=-1
  Data Type Conversion{1,3,7,10} (4 alike) : DataTypeConversion  OutDataTypeStr=uint16
  Data Type Conversion{2,4..6,8..9,11..12} (8 alike) : DataTypeConversion  OutDataTypeStr=uint8
  Mux : Mux  Inputs=8
  Shift Arithmetic{1..4} (4 alike) : ArithShift  BitShiftNumber=8  BitShiftDirection=Right
  Terminator : Terminator
  wires:
  FL/1 -> Data Type Conversion3/1
  Data Type Conversion3/1 -> Bitwise Operator/1, Bitwise Operator1/1
  Bitwise Operator1/1 -> Shift Arithmetic1/1
  Shift Arithmetic1/1 -> Data Type Conversion4/1
  Bitwise Operator/1 -> Data Type Conversion5/1
  FR/1 -> Data Type Conversion1/1
  Data Type Conversion1/1 -> Bitwise Operator2/1, Bitwise Operator3/1
  Bitwise Operator3/1 -> Shift Arithmetic2/1
  Shift Arithmetic2/1 -> Data Type Conversion2/1
  Bitwise Operator2/1 -> Data Type Conversion6/1
  RL/1 -> Data Type Conversion7/1
  Data Type Conversion7/1 -> Bitwise Operator4/1, Bitwise Operator5/1
  Bitwise Operator5/1 -> Shift Arithmetic3/1
  Shift Arithmetic3/1 -> Data Type Conversion8/1
  Bitwise Operator4/1 -> Data Type Conversion9/1
  RR/1 -> Data Type Conversion10/1
  Data Type Conversion10/1 -> Bitwise Operator6/1, Bitwise Operator7/1
  Bitwise Operator7/1 -> Shift Arithmetic4/1
  Shift Arithmetic4/1 -> Data Type Conversion11/1
  Bitwise Operator6/1 -> Data Type Conversion12/1
  Data Type Conversion12/1 -> Mux/8
  Data Type Conversion11/1 -> Mux/7
  Data Type Conversion9/1 -> Mux/6
  Data Type Conversion8/1 -> Mux/5
  Data Type Conversion6/1 -> Mux/4
  Data Type Conversion2/1 -> Mux/3
  Data Type Conversion5/1 -> Mux/2
  Data Type Conversion4/1 -> Mux/1
  Mux/1 -> CANTransmit/1
  CANTransmit/1 -> Terminator/1  "CAN0522OK_mea"

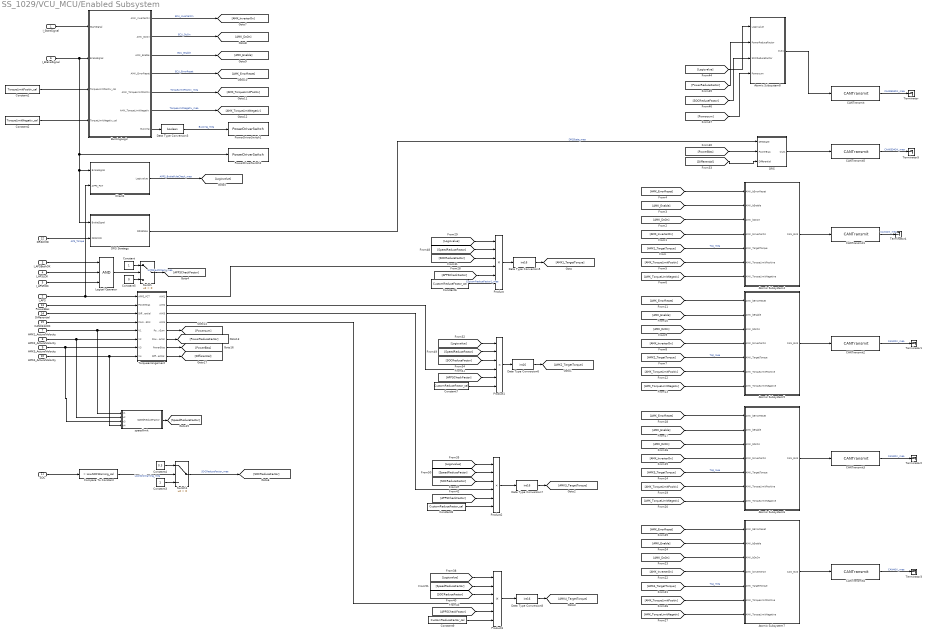
== system SS_1029/VCU_MCU/Enabled Subsystem ==
  I_StartSignal : Inport
  I_APS : Inport  Port=2
  I_APSBothOK : Inport  Port=3
  I_APSLOK : Inport  Port=4
  I_APSROK : Inport  Port=5
  I_BrakeSignal : Inport  Port=6
  AMK1_ActuralVelocity : Inport  Port=7
  AMK2_ActuralVelocity : Inport  Port=8
  AMK3_ActuralVelocity : Inport  Port=9
  AMK4_ActuralVelocity : Inport  Port=10
  SOC : Inport  Port=11
  DRSCMD : Inport  Port=12
  PowerBias : Inport  Port=13
  Differential : Inport  Port=14
  CAN0333OK : Inport  Port=15
  Atomic Subsystem4 : Subsystem  TreatAsAtomicUnit=on
  Atomic Subsystem5 : Subsystem  TreatAsAtomicUnit=on
  Atomic Subsystem6 : Subsystem  TreatAsAtomicUnit=on
  Atomic Subsystem7 : Subsystem  TreatAsAtomicUnit=on
  Atomic Subsystem8 : Subsystem  TreatAsAtomicUnit=on
  BuzzingLogic : Stateflow chart  TreatAsAtomicUnit=on
  CANTransmit : ec55xxlib/RapidECU_U2/07CANCommucation/CANTransmit  canmodule=B  canbuffer=58  canmessageid=hex2dec('0518')  canmessagetype=Standard(11-bit ID)  datalength=8  sampletime=-1
  CANTransmit1 : ec55xxlib/RapidECU_U2/07CANCommucation/CANTransmit  canmodule=A  canbuffer=8  canmessageid=hex2dec('0184')  canmessagetype=Standard(11-bit ID)  datalength=8  sampletime=-1
  CANTransmit2 : ec55xxlib/RapidECU_U2/07CANCommucation/CANTransmit  canmodule=A  canbuffer=9  canmessageid=hex2dec('0185')  canmessagetype=Standard(11-bit ID)  datalength=8  sampletime=-1
  CANTransmit3 : ec55xxlib/RapidECU_U2/07CANCommucation/CANTransmit  canmodule=A  canbuffer=10  canmessageid=hex2dec('0188')  canmessagetype=Standard(11-bit ID)  datalength=8  sampletime=-1
  CANTransmit4 : ec55xxlib/RapidECU_U2/07CANCommucation/CANTransmit  canmodule=A  canbuffer=11  canmessageid=hex2dec('0189')  canmessagetype=Standard(11-bit ID)  datalength=8  sampletime=-1
  CANTransmit5 : ec55xxlib/RapidECU_U2/07CANCommucation/CANTransmit  canmodule=B  canbuffer=60  canmessageid=hex2dec('0334')  canmessagetype=Standard(11-bit ID)  datalength=8  sampletime=-1
  Chart1 : Stateflow chart  TreatAsAtomicUnit=on
  Compare To Constant : simulink/Logic and Bit Operations/Compare To Constant  relop=<  const=LowSOCWarning_cal  OutDataTypeStr=boolean
  Constant : Constant  OutDataTypeStr=single  SampleTime=-1
  Constant1 : Constant  Value=TorqueLimitPositiv_cal  OutDataTypeStr=int16  SampleTime=-1
  Constant2 : Constant  Value=TorqueLimitNegativ_cal  OutDataTypeStr=int16  SampleTime=-1
  Constant3 : Constant  OutDataTypeStr=single  SampleTime=-1
  Constant4 : Constant  Value=0.3  OutDataTypeStr=single  SampleTime=-1
  Constant5 : Constant  Value=0  OutDataTypeStr=single  SampleTime=-1
  Constant{6..9} (4 alike) : Constant  Value=CustomReduceFactor_cal  OutDataTypeStr=single  SampleTime=-1
  DRS : Subsystem  TreatAsAtomicUnit=on
  DRS Strategy : Stateflow chart  TreatAsAtomicUnit=on
  Data Type Conversion3 : DataTypeConversion  OutDataTypeStr=boolean
  Data Type Conversion{5..8} (4 alike) : DataTypeConversion  OutDataTypeStr=int16
  Logical Operator : Logic  Inputs=3  AllPortsSameDT=off  OutDataTypeStr=boolean
  PowerDriverSwitch1 : ec55xxlib/RapidECU_U2/04PowerDriverSwitch/PowerDriverSwitch  channel=114: O_PWM9_HS2A9  sampletime=-1
  PowerDriverSwitch2 : ec55xxlib/RapidECU_U2/04PowerDriverSwitch/PowerDriverSwitch  channel=115: O_PWM10_HS2A9  sampletime=-1
  Product{,1..3} (4 alike) : Product  Inputs=6  OutDataTypeStr=single
  Switch : Switch  Criteria=u2 > Threshold
  Switch1 : Switch  Criteria=u2 > Threshold
  Terminator{,1..5} (6 alike) : Terminator
  Torquearrengement : Subsystem  TreatAsAtomicUnit=on
  "speedlimit " : Subsystem
  wires:
  CANTransmit1/1 -> Terminator4/1  "CAN1OK_mea"
  I_APS/1 -> Torquearrengement/1(APPS_PCT), Chart1/2(APPS_PCT)  "APS_Torque"
  CANTransmit2/1 -> Terminator1/1  "CAN2OK_mea"
  CANTransmit3/1 -> Terminator2/1  "CAN3OK_mea"
  CANTransmit4/1 -> Terminator3/1  "CAN4OK_mea"
  I_BrakeSignal/1 -> DRS Strategy/1(BrakeSignal), Chart1/1(BrakeSignal), PowerDriverSwitch2/1, BuzzingLogic/2(BrakeSignal)
  I_StartSignal/1 -> BuzzingLogic/1(StartSignal)
  Constant1/1 -> BuzzingLogic/3(TorqueLimitPositiv_cal)
  Constant2/1 -> BuzzingLogic/4(TorqueLimitNegativ_cal)
  BuzzingLogic/7(Buzzing) -> Data Type Conversion3/1
  Data Type Conversion3/1 -> PowerDriverSwitch1/1  "Buzzing_mea"
  BuzzingLogic/1(AMK_InverterOn) -> [AMK_InverterOn]  "ECU_InverterOn"
  BuzzingLogic/2(AMK_DcOn) -> [AMK_DcOn]  "ECU_DcOn"
  BuzzingLogic/4(AMK_ErrorReset) -> [AMK_ErrorReset]  "ECU_ErrorReset"
  BuzzingLogic/5(AMK_TorqueLimitPositiv) -> [AMK_TorqueLimitPositiv]  "TorqueLimitPositiv_mea"
  BuzzingLogic/6(AMK_TorqueLimitNegativ) -> [AMK_TorqueLimitNegativ]  "TorqueLimitNegativ_mea"
  AMK4_ActuralVelocity/1 -> "speedlimit "/4(v4), Torquearrengement/8(V4)
  I_APSLOK/1 -> Logical Operator/2
  I_APSROK/1 -> Logical Operator/3
  I_APSBothOK/1 -> Logical Operator/1
  BuzzingLogic/3(AMK_Enable) -> [AMK_Enable]  "ECU_Enable"
  Logical Operator/1 -> Switch/2
  Product/1 -> Data Type Conversion5/1
  Data Type Conversion5/1 -> [AMK1_TargetTorque]
  Atomic Subsystem4/1(CAN_BUS) -> CANTransmit1/1
  [AMK_ErrorReset] -> Atomic Subsystem4/1(AMK_bErrorReset)
  [AMK_Enable] -> Atomic Subsystem4/2(AMK_bEnable)
  [AMK_DcOn] -> Atomic Subsystem4/3(AMK_bDcOn)
  [AMK_InverterOn] -> Atomic Subsystem4/4(AMK_bInverterOn)
  [AMK1_TargetTorque] -> Atomic Subsystem4/5(AMK_TargetTorque)  "Tq1_mea"
  [AMK_TorqueLimitPositiv] -> Atomic Subsystem4/6(AMK_TorqueLimitPositive)
  [AMK_TorqueLimitNegativ] -> Atomic Subsystem4/7(AMK_TorqueLimitNegative)
  [AMK_ErrorReset] -> Atomic Subsystem5/1(AMK_bErrorReset)
  [AMK_Enable] -> Atomic Subsystem5/2(AMK_bEnable)
  [AMK_DcOn] -> Atomic Subsystem5/3(AMK_bDcOn)
  [AMK_InverterOn] -> Atomic Subsystem5/4(AMK_bInverterOn)
  [AMK2_TargetTorque] -> Atomic Subsystem5/5(AMK_TargetTorque)  "Tq2_mea"
  [AMK_TorqueLimitPositiv] -> Atomic Subsystem5/6(AMK_TorqueLimitPositive)
  [AMK_TorqueLimitNegativ] -> Atomic Subsystem5/7(AMK_TorqueLimitNegative)
  [AMK_ErrorReset] -> Atomic Subsystem6/1(AMK_bErrorReset)
  [AMK_Enable] -> Atomic Subsystem6/2(AMK_bEnable)
  [AMK_DcOn] -> Atomic Subsystem6/3(AMK_bDcOn)
  [AMK_InverterOn] -> Atomic Subsystem6/4(AMK_bInverterOn)
  [AMK3_TargetTorque] -> Atomic Subsystem6/5(AMK_TargetTorque)  "Tq3_mea"
  [AMK_TorqueLimitPositiv] -> Atomic Subsystem6/6(AMK_TorqueLimitPositive)
  [AMK_TorqueLimitNegativ] -> Atomic Subsystem6/7(AMK_TorqueLimitNegative)
  [AMK_ErrorReset] -> Atomic Subsystem7/1(AMK_bErrorReset)
  [AMK_Enable] -> Atomic Subsystem7/2(AMK_bEnable)
  [AMK_DcOn] -> Atomic Subsystem7/3(AMK_bDcOn)
  [AMK_InverterOn] -> Atomic Subsystem7/4(AMK_bInverterOn)
  [AMK4_TargetTorque] -> Atomic Subsystem7/5(AMK_TargetTorque)  "Tq4_mea"
  [AMK_TorqueLimitPositiv] -> Atomic Subsystem7/6(AMK_TorqueLimitPositive)
  [AMK_TorqueLimitNegativ] -> Atomic Subsystem7/7(AMK_TorqueLimitNegative)
  Atomic Subsystem7/1(CAN_BUS) -> CANTransmit4/1
  Atomic Subsystem6/1(CAN_BUS) -> CANTransmit3/1
  Atomic Subsystem5/1(CAN_BUS) -> CANTransmit2/1
  SOC/1 -> Compare To Constant/1
  Compare To Constant/1 -> Switch1/2  "LowSOCWarning_mea"
  Constant3/1 -> Switch1/3
  Constant4/1 -> Switch1/1
  Switch1/1 -> [SOCReduceFactor]  "SOCReduceFactor_mea"
  Chart1/1(Logicvalue) -> [Logicvalue]  "APPS_BrakeRuleCheck_mea"
  [SOCReduceFactor] -> Product/3
  [Logicvalue] -> Product/1
  Product1/1 -> Data Type Conversion6/1
  Data Type Conversion6/1 -> [AMK2_TargetTorque]
  [SOCReduceFactor] -> Product1/3
  [Logicvalue] -> Product1/1
  Product2/1 -> Data Type Conversion7/1
  Data Type Conversion7/1 -> [AMK3_TargetTorque]
  [SOCReduceFactor] -> Product2/3
  [Logicvalue] -> Product2/1
  Product3/1 -> Data Type Conversion8/1
  Data Type Conversion8/1 -> [AMK4_TargetTorque]
  [SOCReduceFactor] -> Product3/3
  [Logicvalue] -> Product3/1
  Constant/1 -> Switch/1
  Constant5/1 -> Switch/3
  Switch/1 -> [APPSCheckFactor]  "APPSFaultCheck_mea"
  [APPSCheckFactor] -> Product/5
  [APPSCheckFactor] -> Product1/5
  [APPSCheckFactor] -> Product2/5
  [APPSCheckFactor] -> Product3/5
  [Powersum] -> Atomic Subsystem8/4(Powersum)
  [SOCReduceFactor] -> Atomic Subsystem8/3(SOCReduceFactor)
  [PowerReduceFactor] -> Atomic Subsystem8/2(PowerReduceFactor)
  [Logicvalue] -> Atomic Subsystem8/1(Logicvalue)
  Constant6/1 -> Product/6  "CustomReduceFactor1_mea"
  Constant7/1 -> Product1/6
  Constant8/1 -> Product2/6
  Constant9/1 -> Product3/6
  DRSCMD/1 -> DRS Strategy/2(DRSCMD)
  DRS Strategy/1(DRSState) -> DRS/1(DRSState)  "DRSState_mea"
  [SpeedReduceFactor] -> Product/2
  [SpeedReduceFactor] -> Product1/2
  [SpeedReduceFactor] -> Product2/2
  [SpeedReduceFactor] -> Product3/2
  CANTransmit/1 -> Terminator/1  "CAN0518OK_mea"
  Atomic Subsystem8/1(Out1) -> CANTransmit/1
  DRS/1(Out1) -> CANTransmit5/1
  CANTransmit5/1 -> Terminator5/1  "CAN0334OK_mea"
  AMK1_ActuralVelocity/1 -> Torquearrengement/5(V1), "speedlimit "/1(v1)
  AMK3_ActuralVelocity/1 -> "speedlimit "/3(v3), Torquearrengement/7(V3)
  "speedlimit "/1(SpeedReduceFactor) -> [SpeedReduceFactor]
  AMK2_ActuralVelocity/1 -> "speedlimit "/2(v2), Torquearrengement/6(V2)
  Torquearrengement/1(AIM1) -> Product/4
  Torquearrengement/2(AIM2) -> Product1/4
  Torquearrengement/3(AIM3) -> Product2/4
  Torquearrengement/4(AIM4) -> Product3/4
  Torquearrengement/6(PowerReduceFactor) -> [PowerReduceFactor]
  Torquearrengement/5(PowerSum) -> [Powersum]
  PowerBias/1 -> Torquearrengement/2(PowerBias)
  Differential/1 -> Torquearrengement/3(Differential)
  CAN0333OK/1 -> Torquearrengement/4(CAN0333OK)
  Torquearrengement/7("PowerBias ") -> [PowerBias]
  Torquearrengement/8("Differential ") -> [Differential]
  [PowerBias] -> DRS/2(PowerBias)
  [Differential] -> DRS/3("Differential ")

== system SS_1029/HardWare_Input/BMS Info/Subsystem ==
  "Enable " : Inport
  CANMsg : Inport  Port=2
  function : TriggerPort  TriggerType=function-call
  Subsystem : Subsystem
  Voltage_MSB : Outport
  Voltage_LSB : Outport  Port=2
  SOC : Outport  Port=3
  wires:
  CANMsg/1 -> Subsystem/1(CANMsg)
  Subsystem/1(Voltage_MSB) -> Voltage_MSB/1
  Subsystem/2(Voltage_LSB) -> Voltage_LSB/1
  Subsystem/3(SOC) -> SOC/1
  "Enable "/1 -> Subsystem/Enable

== system SS_1029/HardWare_Input/DRS CMDInput/Subsystem ==
  Enable : Inport
  CANMsg : Inport  Port=2
  function : TriggerPort  TriggerType=function-call
  Subsystem : Subsystem
  DRS : Outport
  PowerBias : Outport  Port=2
  Differential : Outport  Port=3
  wires:
  CANMsg/1 -> Subsystem/1(CANMsg)
  Subsystem/1(DRS) -> DRS/1
  Enable/1 -> Subsystem/Enable
  Subsystem/2(PowerBias) -> PowerBias/1
  Subsystem/3(Differential) -> Differential/1

== system SS_1029/HardWare_Input/In1_Message/Function-Call Subsystem ==
  Enable : Inport
  CANMsg : Inport  Port=2
  function : TriggerPort  TriggerType=function-call
  Subsystem1 : Subsystem
  AMK_ActuralVelocity : Outport
  AMK_ActuralTorque : Outport  Port=2
  AMK_bSystemReady : Outport  Port=3
  AMK_bError : Outport  Port=4
  AMK_bQuitDcOn : Outport  Port=5
  "AMK_bQuitInverterOn " : Outport  Port=6
  wires:
  CANMsg/1 -> Subsystem1/1(In1)
  Subsystem1/1(Out1) -> AMK_bSystemReady/1
  Subsystem1/2(Out2) -> AMK_bError/1
  Subsystem1/3(Out3) -> AMK_bQuitDcOn/1
  Subsystem1/4(Out4) -> "AMK_bQuitInverterOn "/1
  Subsystem1/5(Out5) -> AMK_ActuralVelocity/1
  Subsystem1/6(Out6) -> AMK_ActuralTorque/1
  Enable/1 -> Subsystem1/Enable
